simulink model "bloques_PD"  (R2021b)
settings: Solver=FixedStepAuto  StartTime=0.0  StopTime=Tc  FixedStep=Ts  RelTol=1e-3
values from neighbouring files (symbols this model uses):
  a = 210.90461*(Ts*Ts)    (= 2.1090461e-06)    [raiz.m]
  b = 25.65696*Ts - 2.0    (= -1.997434304)    [raiz.m]
  c = 1.0 - 25.65696*Ts + 210.90461*(Ts*Ts)    (= 0.997436413046)    [raiz.m]
  e = 2.14036*(Ts*Ts)    (= 2.14036e-08)    [raiz.m]
  g1 = kp + (kd/Tz)    (= 748.90662)    [raiz.m]
  g2 = kd/Tz    (= 745.675)    [raiz.m]
  limit = 46    [raiz.m]
  sp = 0.0    (= 0)    [raiz.m]
  Tz = 0.002    [raiz.m]
settings Model: Creator=yeezvs  LastModifiedBy=yeezvs
settings DataIOCC: ReturnWorkspaceOutputs=off

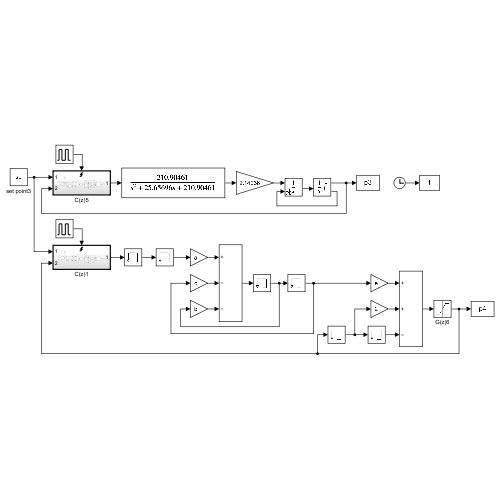
[thumbnail: Simulink's stored preview of the top-level diagram]
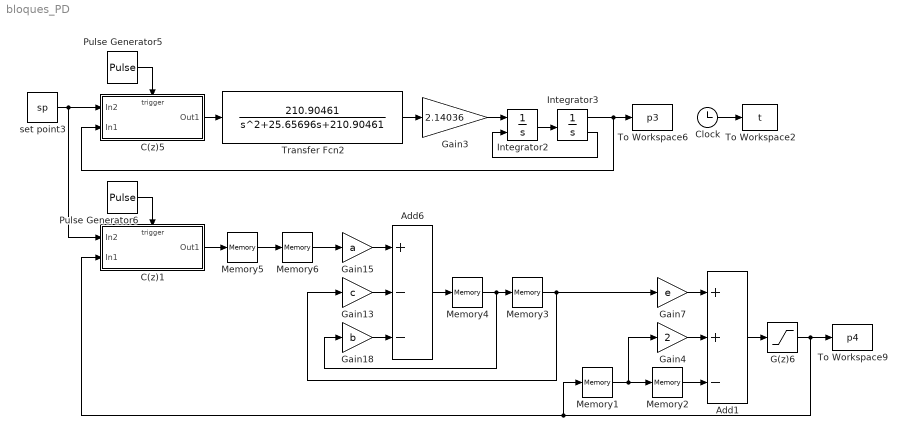
== system bloques_PD ==
  Add1 : Sum  Inputs=++-
  Add6 : Sum  Inputs=+--
  C(z)1 : Subsystem  TreatAsAtomicUnit=on
  C(z)5 : Subsystem  TreatAsAtomicUnit=on
  Clock : Clock
  G(z)6 : Saturate  UpperLimit=0.15  LowerLimit=-0.15
  Gain13 : Gain  Gain=c
  Gain15 : Gain  Gain=a
  Gain18 : Gain  Gain=b
  Gain3 : Gain  Gain=2.14036
  Gain4 : Gain  Gain=2
  Gain7 : Gain  Gain=e
  Integrator2 : Integrator  ExternalReset=either
  Integrator3 : Integrator  InitialCondition=0.15  LimitOutput=on  UpperSaturationLimit=0.15  LowerSaturationLimit=-0.15  ShowSaturationPort=on
  Memory1 : Memory  InitialCondition=0.15
  Memory2 : Memory  InitialCondition=0.15
  Memory{3..6} (4 alike) : Memory
  Pulse Generator5 : DiscretePulseGenerator  PulseType=Time based  Period=Tz  PulseWidth=50
  Pulse Generator6 : DiscretePulseGenerator  PulseType=Time based  Period=Tz  PulseWidth=50
  To Workspace2 : ToWorkspace  VariableName=t  SampleTime=-1
      settings: Save2DSignal=2-D array (concatenate along first dimension)
  To Workspace6 : ToWorkspace  VariableName=p3  SampleTime=-1
      settings: Save2DSignal=2-D array (concatenate along first dimension)
  To Workspace9 : ToWorkspace  VariableName=p4  SampleTime=-1
      settings: Save2DSignal=2-D array (concatenate along first dimension)
  Transfer Fcn2 : TransferFcn  Numerator=[210.90461]  Denominator=[1 25.65696 210.90461]
  set point3 : Constant  Value=sp
  wires:
  Gain7/1 -> Add1/1
  Add1/1 -> G(z)6/1
  Memory1/1 -> Gain4/1, Memory2/1
  Pulse Generator6/1 -> C(z)1/Trigger
  Memory5/1 -> Memory6/1
  Gain4/1 -> Add1/2
  Gain13/1 -> Add6/2
  Gain15/1 -> Add6/1
  C(z)1/1(Out1) -> Memory5/1
  Gain18/1 -> Add6/3
  Transfer Fcn2/1 -> Gain3/1
  Memory2/1 -> Add1/3
  G(z)6/1 -> To Workspace9/1, C(z)1/2(In1), Memory1/1
  Add6/1 -> Memory4/1
  Integrator3/1 -> To Workspace6/1, C(z)5/2(In1)
  Memory3/1 -> Gain7/1, Gain13/1
  Pulse Generator5/1 -> C(z)5/Trigger
  Memory6/1 -> Gain15/1
  C(z)5/1(Out1) -> Transfer Fcn2/1
  set point3/1 -> C(z)1/1(In2), C(z)5/1(In2)
  Memory4/1 -> Memory3/1, Gain18/1
  Integrator3/2 -> Integrator2/2
  Gain3/1 -> Integrator2/1
  Integrator2/1 -> Integrator3/1
  Clock/1 -> To Workspace2/1

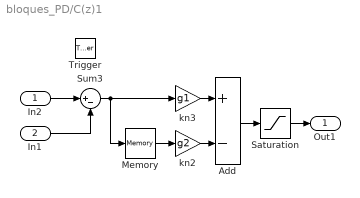
== system bloques_PD/C(z)1 ==
  In2 : Inport
  In1 : Inport  Port=2
  Trigger : TriggerPort  VariantControl=(inherit)
  Add : Sum  Inputs=+-
  Memory : Memory  InheritSampleTime=on
  Saturation : Saturate  UpperLimit=limit  LowerLimit=-limit
  Sum3 : Sum  Inputs=|+-
  kn2 : Gain  Gain=g2
  kn3 : Gain  Gain=g1
  Out1 : Outport
  wires:
  In2/1 -> Sum3/1
  In1/1 -> Sum3/2
  kn3/1 -> Add/1
  kn2/1 -> Add/2
  Memory/1 -> kn2/1
  Sum3/1 -> kn3/1, Memory/1
  Add/1 -> Saturation/1
  Saturation/1 -> Out1/1

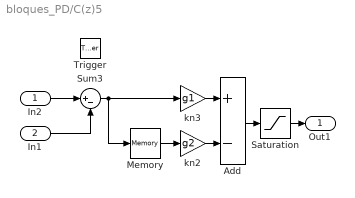
== system bloques_PD/C(z)5 ==
  In2 : Inport
  In1 : Inport  Port=2
  Trigger : TriggerPort  VariantControl=(inherit)
  Add : Sum  Inputs=+-
  Memory : Memory  InheritSampleTime=on
  Saturation : Saturate  UpperLimit=limit  LowerLimit=-limit
  Sum3 : Sum  Inputs=|+-
  kn2 : Gain  Gain=g2
  kn3 : Gain  Gain=g1
  Out1 : Outport
  wires:
  In2/1 -> Sum3/1
  In1/1 -> Sum3/2
  kn3/1 -> Add/1
  kn2/1 -> Add/2
  Memory/1 -> kn2/1
  Sum3/1 -> kn3/1, Memory/1
  Add/1 -> Saturation/1
  Saturation/1 -> Out1/1
